simulink library "INT_Tra_Los"  (R2016b)
settings: Solver=VariableStepAuto  StartTime=0.0  StopTime=10.0  RelTol=1e-3
settings Model: Creator=Administrator  LastModifiedBy=Administrator

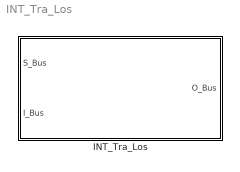
== system INT_Tra_Los ==
  INT_Tra_Los : Subsystem

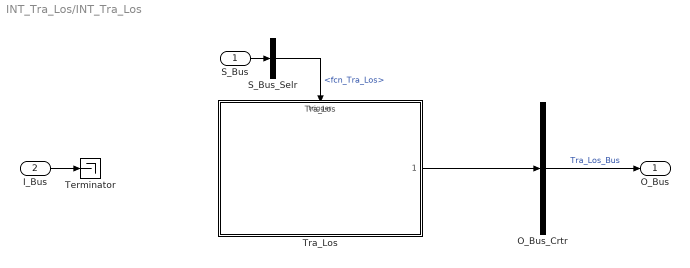
== system INT_Tra_Los/INT_Tra_Los ==
  S_Bus : Inport
  I_Bus : Inport  Port=2
  O_Bus_Crtr : BusCreator  Inputs=1
  S_Bus_Selr : BusSelector  OutputSignals=fcn_Tra_Los
  Terminator : Terminator
  Tra_Los : ModelReference  ModelNameDialog=Tra_Los  SimulationMode=Normal  ModelReferenceVersion=1.10  TriggerPortName=function  TriggerPortTriggerType=function-call  TriggerPortStatesWhenEnabling=held
  O_Bus : Outport
  wires:
  S_Bus_Selr/1 -> Tra_Los/Trigger  "<fcn_Tra_Los>"
  S_Bus/1 -> S_Bus_Selr/1
  I_Bus/1 -> Terminator/1
  O_Bus_Crtr/1 -> O_Bus/1  "Tra_Los_Bus"
  Tra_Los/1 -> O_Bus_Crtr/1
